simulink model "full_maneuver_single_veh"  (R2020a)
settings: Solver=VariableStepAuto  StartTime=0.0  StopTime=90  FixedStep=0.1  MaxStep=5e-2  RelTol=1e-3
InitFcn:
  | totalVehicles = 5;
  | if exist('vehStatesBus', 'var')==0
  | load vehBuses
  | end
  | if exist('vehErrorsBus', 'var')==0
  | load vehBuses
  | end
libraries: simulink x69, powerlib_meascontrol x6, autolibshared x6, dspsigops x3, eeGeneralControl x2
(part 1 of 6)
settings Model: Creator=fvall  LastModifiedBy=fvall
settings SFSimCC: CustomCodeUndefinedFunction=UseInterfaceOnly

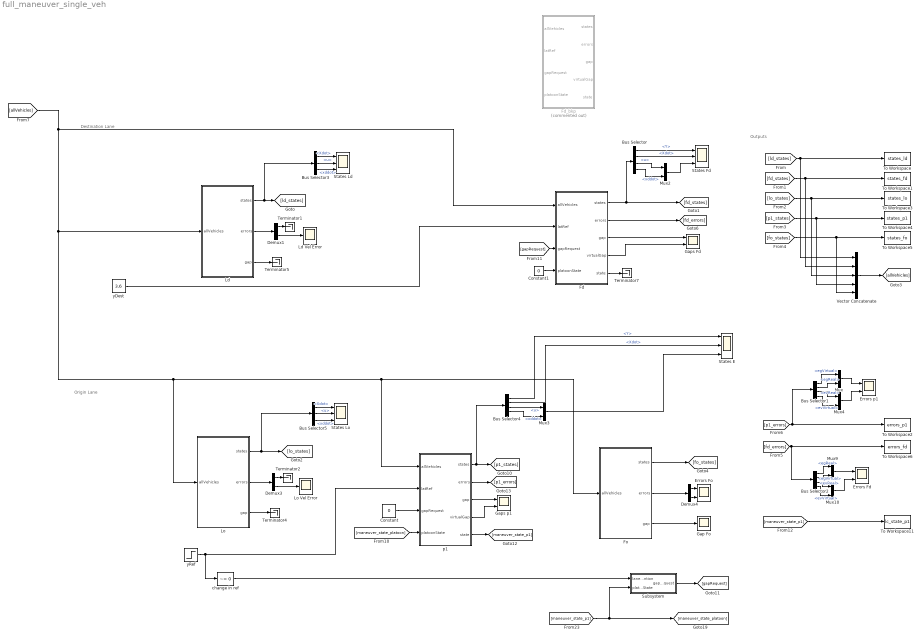
== system full_maneuver_single_veh ==
  note: Destination Lane
  note: Outputs
  note: Origin Lane
  Bus Selector : BusSelector  OutputSignals=Y,Xdot,u,xddot
  Bus Selector1 : BusSelector  OutputSignals=egVirtual,egReal,evReal,evVirtual
  Bus Selector2 : BusSelector  OutputSignals=egReal,egVirtual,evReal,evVirtual
  Bus Selector3 : BusSelector  OutputSignals=Xdot,u,xddot
  Bus Selector4 : BusSelector  OutputSignals=Y,Xdot,u,xddot
  Bus Selector5 : BusSelector  OutputSignals=Xdot,u,xddot
  Constant : Constant  Value=0
  Constant1 : Constant  Value=0
  Demux1 : Demux  Outputs=2
  Demux3 : Demux  Outputs=2
  Demux4 : Demux  Outputs=2
  Errors Fd : Scope  NumInputPorts=2
  Errors Fo : Scope  NumInputPorts=2
  Errors p1 : Scope  NumInputPorts=2
  Fd : Subsystem  mask{m=2000, lf=2.5, lr=2.5, maxAcceleration=3, minAcceleration=-8, maxJerk=50, minJerk=-50, maxDelta=0.43633, maxDeltaDot=0.16406, freeFlowVel=30, posInPlatoon=1, tau=0.5, A=[0 1 15 0;0 -3.06666666666667 0 -16.8666666666667;0 0 0 1;0 -0.933333333333333 0 -10.1333333333333], B=[0;24;0;36], C=[1 0 0 0;0 1 0 0;0 0 1 0;0 0 0 1], x0=24.5938, vx0=15, y0=3.6, h=0.56375, d0=0.5, minGapError=-100, maxGapError=Inf, velFilterGain=10, Kd=1.7738, Kp=0.17738, Ki=0, Ka=0.97561, Kdd=0.097561, velKi=0.0047047, velKp=0.093693, velKd=-0.53954, hFilterGain=1, hFilterSaturation=0.5, vMin=9.75, maxComfAccel=0.6, minComfAccel=-0.4, maxComfJerk=10, minComfJerk=-10, strategy=1, hLC=1.3256, d0LC=0.5, Klat=[0.0363636363636363 -0.0124557881655676 0.972727272727275 0.00274830322149061], L=[3 1 15 0;0 2.93333333333333 0 -16.8666666666667;0 0 12 1;0 -0.933333333333333 0 7.86666666666667]}
      mask prompts: m "autoblks_shared:autoblkVehBody3DofLat:blkPrm_m"; lf "autoblks_shared:autoblkVehBody3DofLat:blkPrm_a"; lr "autoblks_shared:autoblkVehBody3DofLat:blkPrm_b"; maxAcceleration "Max Acceleration"; minAcceleration "Min Acceleration"; maxJerk "Max Jerk"; minJerk "Min Jerk"; maxDelta "Max Delta"; maxDeltaDot "Max Delta Dot"; freeFlowVel "Free Flow Velocity"; posInPlatoon "Position in Platoon"; tau "Actuator Lag"; x0 "autoblks_shared:autoblkVehBody3DofLat:blkPrm_X_o"; vx0 "autoblks_shared:autoblkVehBody3DofLat:blkPrm_xdot_o"; y0 "autoblks_shared:autoblkVehBody3DofLat:blkPrm_Y_o"; h "Time Headway"; d0 "Standstill Gap"; minGapError "Min Gap Error"; maxGapError "Max Gap Error"; velFilterGain "Velocity Filter Gain"; hFilterGain "Headway Filter Gain"; hFilterSaturation "Headway Filter Saturation"; vMin "Min Velocity"; maxComfAccel "Max Comf Accel"; minComfAccel "Min Comf Accel"; maxComfJerk "Max Comf Jerk"; minComfJerk "Min Comf Jerk"; strategy "LC strategy"; hLC "Time Headway LC"; d0LC "Standstill Gap LC"; Klat "Lat Controller Gain"; L "Observer Gain"
      mask TypeOptions m: Vehicle Body 3DOF Single Track/m
      mask TypeOptions lf: Vehicle Body 3DOF Single Track/a
      mask TypeOptions lr: Vehicle Body 3DOF Single Track/b
      mask TypeOptions maxDelta: Lateral Control/Saturation/UpperLimit
      mask TypeOptions maxDeltaDot: Lateral Control/Rate Limiter/RisingSlewLimit
      mask TypeOptions posInPlatoon: posInPlatoon/Value
      mask TypeOptions A:
      | Lateral Control/Full State
      | Observer/Gain3/Gain
      mask TypeOptions B:
      | Lateral Control/Full State
      | Observer/Gain/Gain
      mask TypeOptions C:
      | Lateral Control/Full State
      | Observer/Gain1/Gain
      mask TypeOptions x0: Vehicle Body 3DOF Single Track/X_o
      mask TypeOptions vx0: Vehicle Body 3DOF Single Track/xdot_o
      mask TypeOptions y0: Vehicle Body 3DOF Single Track/Y_o
      mask TypeOptions strategy: strategy/Value
      mask TypeOptions Klat: Lateral Control/Gain1/Gain
      mask TypeOptions L:
      | Lateral Control/Full State
      | Observer/Gain2/Gain
      mask DialogControl DescGroupVar Prompt: 3DOF Vehicle with ACC
      mask DialogControl DescTextVar Prompt: Vehicle with ACC. The vehicle model is Simulink's 3DOF single track vehicle body. The controller is a PID with constant headway including headway error saturation and filtered leader velocity.
      mask DialogControl VehParams Prompt: Vehicle Parameters
      mask DialogControl m Prompt: Vehicle mass, m [kg]:
      mask DialogControl lf Prompt: Longitudinal distance from center of mass to front axle, a [m]:
      mask DialogControl lr Prompt: Longitudinal distance from center of mass to rear axle, b [m]:
      mask DialogControl latLinearModel Prompt: Lat Linear Model
      mask DialogControl InitStates Prompt: Initial State
      mask DialogControl x0 Prompt: Initial inertial frame longitudinal position, X_o [m]:
      mask DialogControl vx0 Prompt: Initial longitudinal velocity, xdot_o [m/s]:
      mask DialogControl y0 Prompt: Initial inertial frame lateral displacement, Y_o [m]:
      mask DialogControl Container3 Prompt: Veh Following Parameters
      mask DialogControl ComfortConstraints Prompt: Comfort Constraints
      mask DialogControl LCParams Prompt: Lane Change Params
  Fd_bkp : Subsystem  Commented=on  mask{m=2000, lf=2.5, lr=2.5, maxAcceleration=3, minAcceleration=-8, maxJerk=50, minJerk=-50, maxDelta=0.43633, maxDeltaDot=0.16406, freeFlowVel=30, posInPlatoon=1, tau=0.5, A=[0 1 20 0;0 -2.3 0 -21.4;0 0 0 1;0 -0.7 0 -7.6], B=[0;24;0;36], C=[1 0 0 0;0 1 0 0;0 0 1 0;0 0 0 1], x0=-6.2192, vx0=25, y0=3.6, h=0.56375, d0=0.32452, minHeadwayError=-100, maxHeadwayError=Inf, velFilterGain=10, Kd=1.7738, Kp=0.17738, Ki=0, Ka=0.97561, Kdd=0.097561, velKi=0.0019848, velKp=0.052702, velKd=-0.65465, hFilterGain=1, hFilterSaturation=0.5, vMin=16.25, maxComfAccel=0.6, minComfAccel=-0.4, maxComfJerk=10, minComfJerk=-10, strategy=1, hLC=1.9506, d0LC=0.32452, Klat=[0.0363636363636331 0.000980533179898461 1.32121212121203 0.0854574223245029], L=[3 1 20 0;0 3.7 0 -21.4;0 0 12 1;0 -0.7 0 10.4]}
      mask prompts: m "autoblks_shared:autoblkVehBody3DofLat:blkPrm_m"; lf "autoblks_shared:autoblkVehBody3DofLat:blkPrm_a"; lr "autoblks_shared:autoblkVehBody3DofLat:blkPrm_b"; maxAcceleration "Max Acceleration"; minAcceleration "Min Acceleration"; maxJerk "Max Jerk"; minJerk "Min Jerk"; maxDelta "Max Delta"; maxDeltaDot "Max Delta Dot"; freeFlowVel "Free Flow Velocity"; posInPlatoon "Position in Platoon"; tau "Actuator Lag"; x0 "autoblks_shared:autoblkVehBody3DofLat:blkPrm_X_o"; vx0 "autoblks_shared:autoblkVehBody3DofLat:blkPrm_xdot_o"; y0 "autoblks_shared:autoblkVehBody3DofLat:blkPrm_Y_o"; h "Time Headway"; d0 "Standstill Gap"; minHeadwayError "Min Headway Error"; maxHeadwayError "Max Headway Error"; velFilterGain "Velocity Filter Gain"; hFilterGain "Headway Filter Gain"; hFilterSaturation "Headway Filter Saturation"; vMin "Min Velocity"; maxComfAccel "Max Comf Accel"; minComfAccel "Min Comf Accel"; maxComfJerk "Max Comf Jerk"; minComfJerk "Min Comf Jerk"; strategy "LC strategy"; hLC "Time Headway LC"; d0LC "Standstill Gap LC"; Klat "Lat Controller Gain"; L "Observer Gain"
      mask TypeOptions m: Vehicle Body 3DOF Single Track/m
      mask TypeOptions lf: Vehicle Body 3DOF Single Track/a
      mask TypeOptions lr: Vehicle Body 3DOF Single Track/b
      mask TypeOptions maxDelta: Lateral Control/Saturation/UpperLimit
      mask TypeOptions maxDeltaDot: Lateral Control/Rate Limiter/RisingSlewLimit
      mask TypeOptions posInPlatoon: posInPlatoon/Value
      mask TypeOptions A:
      | Lateral Control/Full State
      | Observer/Gain3/Gain
      mask TypeOptions B:
      | Lateral Control/Full State
      | Observer/Gain/Gain
      mask TypeOptions C:
      | Lateral Control/Full State
      | Observer/Gain1/Gain
      mask TypeOptions x0: Vehicle Body 3DOF Single Track/X_o
      mask TypeOptions vx0: Vehicle Body 3DOF Single Track/xdot_o
      mask TypeOptions y0: Vehicle Body 3DOF Single Track/Y_o
      mask TypeOptions strategy: strategy/Value
      mask TypeOptions Klat: Lateral Control/Gain1/Gain
      mask TypeOptions L:
      | Lateral Control/Full State
      | Observer/Gain2/Gain
      mask DialogControl DescGroupVar Prompt: 3DOF Vehicle with ACC
      mask DialogControl DescTextVar Prompt: Vehicle with ACC. The vehicle model is Simulink's 3DOF single track vehicle body. The controller is a PID with constant headway including headway error saturation and filtered leader velocity.
      mask DialogControl VehParams Prompt: Vehicle Parameters
      mask DialogControl m Prompt: Vehicle mass, m [kg]:
      mask DialogControl lf Prompt: Longitudinal distance from center of mass to front axle, a [m]:
      mask DialogControl lr Prompt: Longitudinal distance from center of mass to rear axle, b [m]:
      mask DialogControl latLinearModel Prompt: Lat Linear Model
      mask DialogControl InitStates Prompt: Initial State
      mask DialogControl x0 Prompt: Initial inertial frame longitudinal position, X_o [m]:
      mask DialogControl vx0 Prompt: Initial longitudinal velocity, xdot_o [m/s]:
      mask DialogControl y0 Prompt: Initial inertial frame lateral displacement, Y_o [m]:
      mask DialogControl Container3 Prompt: Veh Following Parameters
      mask DialogControl ComfortConstraints Prompt: Comfort Constraints
      mask DialogControl LCParams Prompt: Lane Change Params
  Fo : Subsystem  mask{m=2000, lf=2.5, lr=2.5, maxAcceleration=3, minAcceleration=-8, maxJerk=50, minJerk=-50, freeFlowVel=30, tau=0.5, x0=0, vx0=20, y0=0, h=0.56375, d0=0.5, minGapError=-100, maxGapError=Inf, velFilterGain=10, Kd=1.7738, Kp=0.17738, Ki=0, Ka=0.97561, Kdd=0.097561, velKi=0.0047047, velKp=0.093693, velKd=-0.53954, hFilterGain=1, hFilterSaturation=0.5, vMin=13, maxComfAccel=0.6, minComfAccel=-0.4, maxComfJerk=10, minComfJerk=-10, hLC=1.6381, d0LC=0.5}
      mask prompts: m "autoblks_shared:autoblkVehBody3DofLat:blkPrm_m"; lf "autoblks_shared:autoblkVehBody3DofLat:blkPrm_a"; lr "autoblks_shared:autoblkVehBody3DofLat:blkPrm_b"; maxAcceleration "Max Acceleration"; minAcceleration "Min Acceleration"; maxJerk "Max Jerk"; minJerk "Min Jerk"; freeFlowVel "Free Flow Velocity"; tau "Actuator Lag"; x0 "autoblks_shared:autoblkVehBody3DofLat:blkPrm_X_o"; vx0 "autoblks_shared:autoblkVehBody3DofLat:blkPrm_xdot_o"; y0 "autoblks_shared:autoblkVehBody3DofLat:blkPrm_Y_o"; h "Time Headway"; d0 "Standstill Gap"; minGapError "Min Gap Error"; maxGapError "Max Gap Error"; velFilterGain "Velocity Filter Gain"; hFilterGain "Headway Filter Gain"; hFilterSaturation "Headway Filter Saturation"; vMin "Min Velocity"; maxComfAccel "Max Comf Accel"; minComfAccel "Min Comf Accel"; maxComfJerk "Max Comf Jerk"; minComfJerk "Min Comf Jerk"; hLC "Time Headway LC"; d0LC "Standstill Gap LC"
      mask TypeOptions m: Vehicle Body 3DOF Single Track/m
      mask TypeOptions lf: Vehicle Body 3DOF Single Track/a
      mask TypeOptions lr: Vehicle Body 3DOF Single Track/b
      mask TypeOptions x0: Vehicle Body 3DOF Single Track/X_o
      mask TypeOptions vx0: Vehicle Body 3DOF Single Track/xdot_o
      mask TypeOptions y0: Vehicle Body 3DOF Single Track/Y_o
      mask DialogControl DescGroupVar Prompt: 3DOF Vehicle with ACC
      mask DialogControl DescTextVar Prompt: Vehicle with ACC. The vehicle model is Simulink's 3DOF single track vehicle body. The controller is a PID with constant headway including headway error saturation and filtered leader velocity.
      mask DialogControl VehParams Prompt: Vehicle Parameters
      mask DialogControl m Prompt: Vehicle mass, m [kg]:
      mask DialogControl lf Prompt: Longitudinal distance from center of mass to front axle, a [m]:
      mask DialogControl lr Prompt: Longitudinal distance from center of mass to rear axle, b [m]:
      mask DialogControl InitStates Prompt: Initial State
      mask DialogControl x0 Prompt: Initial inertial frame longitudinal position, X_o [m]:
      mask DialogControl vx0 Prompt: Initial longitudinal velocity, xdot_o [m/s]:
      mask DialogControl y0 Prompt: Initial inertial frame lateral displacement, Y_o [m]:
      mask DialogControl Container3 Prompt: Veh Following Parameters
      mask DialogControl ComfortConstraints Prompt: Comfort Constraints
      mask DialogControl LaneChangeParams Prompt: Lane Change Params
  Gap Fo : Scope
  Gaps Fd : Scope  NumInputPorts=2
  Gaps p1 : Scope  NumInputPorts=2
  Ld : Subsystem  mask{m=2000, lf=2.5, lr=2.5, maxAcceleration=3, minAcceleration=-8, maxJerk=50, minJerk=-50, freeFlowVel=15, tau=0.5, x0=38.55, vx0=15, y0=3.6, h=0.56375, d0=0.5, minGapError=-100, maxGapError=Inf, velFilterGain=10, Kd=1.7738, Kp=0.17738, Ki=0, Ka=0.97561, Kdd=0.097561, velKi=0.0047047, velKp=0.093693, velKd=-0.53954, hFilterGain=1, hFilterSaturation=0.5, vMin=9.75, maxComfAccel=0.6, minComfAccel=-0.4, maxComfJerk=10, minComfJerk=-10, hLC=1.3256, d0LC=0.5}
      mask prompts: m "autoblks_shared:autoblkVehBody3DofLat:blkPrm_m"; lf "autoblks_shared:autoblkVehBody3DofLat:blkPrm_a"; lr "autoblks_shared:autoblkVehBody3DofLat:blkPrm_b"; maxAcceleration "Max Acceleration"; minAcceleration "Min Acceleration"; maxJerk "Max Jerk"; minJerk "Min Jerk"; freeFlowVel "Free Flow Velocity"; tau "Actuator Lag"; x0 "autoblks_shared:autoblkVehBody3DofLat:blkPrm_X_o"; vx0 "autoblks_shared:autoblkVehBody3DofLat:blkPrm_xdot_o"; y0 "autoblks_shared:autoblkVehBody3DofLat:blkPrm_Y_o"; h "Time Headway"; d0 "Standstill Gap"; minGapError "Min Gap Error"; maxGapError "Max Gap Error"; velFilterGain "Velocity Filter Gain"; hFilterGain "Headway Filter Gain"; hFilterSaturation "Headway Filter Saturation"; vMin "Min Velocity"; maxComfAccel "Max Comf Accel"; minComfAccel "Min Comf Accel"; maxComfJerk "Max Comf Jerk"; minComfJerk "Min Comf Jerk"; hLC "Time Headway LC"; d0LC "Standstill Gap LC"
      mask TypeOptions m: Vehicle Body 3DOF Single Track/m
      mask TypeOptions lf: Vehicle Body 3DOF Single Track/a
      mask TypeOptions lr: Vehicle Body 3DOF Single Track/b
      mask TypeOptions x0: Vehicle Body 3DOF Single Track/X_o
      mask TypeOptions vx0: Vehicle Body 3DOF Single Track/xdot_o
      mask TypeOptions y0: Vehicle Body 3DOF Single Track/Y_o
      mask DialogControl DescGroupVar Prompt: 3DOF Vehicle with ACC
      mask DialogControl DescTextVar Prompt: Vehicle with ACC. The vehicle model is Simulink's 3DOF single track vehicle body. The controller is a PID with constant headway including headway error saturation and filtered leader velocity.
      mask DialogControl VehParams Prompt: Vehicle Parameters
      mask DialogControl m Prompt: Vehicle mass, m [kg]:
      mask DialogControl lf Prompt: Longitudinal distance from center of mass to front axle, a [m]:
      mask DialogControl lr Prompt: Longitudinal distance from center of mass to rear axle, b [m]:
      mask DialogControl InitStates Prompt: Initial State
      mask DialogControl x0 Prompt: Initial inertial frame longitudinal position, X_o [m]:
      mask DialogControl vx0 Prompt: Initial longitudinal velocity, xdot_o [m/s]:
      mask DialogControl y0 Prompt: Initial inertial frame lateral displacement, Y_o [m]:
      mask DialogControl Container3 Prompt: Veh Following Parameters
      mask DialogControl ComfortConstraints Prompt: Comfort Constraints
      mask DialogControl LaneChangeParams Prompt: Lane Change Params
  Ld Vel Error : Scope
  Lo : Subsystem  mask{m=2000, lf=2.5, lr=2.5, maxAcceleration=3, minAcceleration=-8, maxJerk=50, minJerk=-50, freeFlowVel=20, tau=0.5, x0=33.55, vx0=20, y0=0, h=0.56375, d0=0.5, minGapError=-100, maxGapError=Inf, velFilterGain=10, Kd=1.7738, Kp=0.17738, Ki=0, Ka=0.97561, Kdd=0.097561, velKi=0.0047047, velKp=0.093693, velKd=-0.53954, hFilterGain=1, hFilterSaturation=0.5, vMin=13, maxComfAccel=0.6, minComfAccel=-0.4, maxComfJerk=10, minComfJerk=-10, hLC=1.6381, d0LC=0.5}
      mask prompts: m "autoblks_shared:autoblkVehBody3DofLat:blkPrm_m"; lf "autoblks_shared:autoblkVehBody3DofLat:blkPrm_a"; lr "autoblks_shared:autoblkVehBody3DofLat:blkPrm_b"; maxAcceleration "Max Acceleration"; minAcceleration "Min Acceleration"; maxJerk "Max Jerk"; minJerk "Min Jerk"; freeFlowVel "Free Flow Velocity"; tau "Actuator Lag"; x0 "autoblks_shared:autoblkVehBody3DofLat:blkPrm_X_o"; vx0 "autoblks_shared:autoblkVehBody3DofLat:blkPrm_xdot_o"; y0 "autoblks_shared:autoblkVehBody3DofLat:blkPrm_Y_o"; h "Time Headway"; d0 "Standstill Gap"; minGapError "Min Gap Error"; maxGapError "Max Gap Error"; velFilterGain "Velocity Filter Gain"; hFilterGain "Headway Filter Gain"; hFilterSaturation "Headway Filter Saturation"; vMin "Min Velocity"; maxComfAccel "Max Comf Accel"; minComfAccel "Min Comf Accel"; maxComfJerk "Max Comf Jerk"; minComfJerk "Min Comf Jerk"; hLC "Time Headway LC"; d0LC "Standstill Gap LC"
      mask TypeOptions m: Vehicle Body 3DOF Single Track/m
      mask TypeOptions lf: Vehicle Body 3DOF Single Track/a
      mask TypeOptions lr: Vehicle Body 3DOF Single Track/b
      mask TypeOptions x0: Vehicle Body 3DOF Single Track/X_o
      mask TypeOptions vx0: Vehicle Body 3DOF Single Track/xdot_o
      mask TypeOptions y0: Vehicle Body 3DOF Single Track/Y_o
      mask DialogControl DescGroupVar Prompt: 3DOF Vehicle with ACC
      mask DialogControl DescTextVar Prompt: Vehicle with ACC. The vehicle model is Simulink's 3DOF single track vehicle body. The controller is a PID with constant headway including headway error saturation and filtered leader velocity.
      mask DialogControl VehParams Prompt: Vehicle Parameters
      mask DialogControl m Prompt: Vehicle mass, m [kg]:
      mask DialogControl lf Prompt: Longitudinal distance from center of mass to front axle, a [m]:
      mask DialogControl lr Prompt: Longitudinal distance from center of mass to rear axle, b [m]:
      mask DialogControl InitStates Prompt: Initial State
      mask DialogControl x0 Prompt: Initial inertial frame longitudinal position, X_o [m]:
      mask DialogControl vx0 Prompt: Initial longitudinal velocity, xdot_o [m/s]:
      mask DialogControl y0 Prompt: Initial inertial frame lateral displacement, Y_o [m]:
      mask DialogControl Container3 Prompt: Veh Following Parameters
      mask DialogControl ComfortConstraints Prompt: Comfort Constraints
      mask DialogControl LaneChangeParams Prompt: Lane Change Params
  Lo Vel Error : Scope
  Mux{,2..4,9..10} (6 alike) : Mux  Inputs=2
  States E : Scope  NumInputPorts=3
  States Fd : Scope  NumInputPorts=3
  States Ld : Scope  NumInputPorts=3
  States Lo : Scope  NumInputPorts=3
  Subsystem : Subsystem
  Terminator{1..2,4..5,7} (5 alike) : Terminator
  To Workspace : ToWorkspace  VariableName=states_ld  SaveFormat=Timeseries  SampleTime=-1
  To Workspace1 : ToWorkspace  VariableName=states_fd  SaveFormat=Timeseries  SampleTime=-1
  To Workspace11 : ToWorkspace  VariableName=lc_state_p1  SaveFormat=Timeseries  SampleTime=-1
  To Workspace2 : ToWorkspace  VariableName=errors_p1  SaveFormat=Timeseries  SampleTime=-1
  To Workspace3 : ToWorkspace  VariableName=states_lo  SaveFormat=Timeseries  SampleTime=-1
  To Workspace4 : ToWorkspace  VariableName=states_p1  SaveFormat=Timeseries  SampleTime=-1
  To Workspace5 : ToWorkspace  VariableName=states_fo  SaveFormat=Timeseries  SampleTime=-1
  To Workspace6 : ToWorkspace  VariableName=errors_fd  SaveFormat=Timeseries  SampleTime=-1
  Vector Concatenate : Concatenate  NumInputs=5
  change in ref : simulink/Logic and Bit Operations/Compare To Constant  relop=~=  const=0  OutDataTypeStr=boolean
  p1 : Subsystem  mask{m=2000, lf=2.5, lr=2.5, maxAcceleration=3, minAcceleration=-8, maxJerk=50, minJerk=-50, maxDelta=0.43633, maxDeltaDot=0.16406, freeFlowVel=30, posInPlatoon=1, tau=0.5, A=[0 1 15 0;0 -3.06666666666667 0 -16.8666666666667;0 0 0 1;0 -0.933333333333333 0 -10.1333333333333], B=[0;24;0;36], C=[1 0 0 0;0 1 0 0;0 0 1 0;0 0 0 1], x0=16.775, vx0=20, y0=0, h=0.56375, d0=0.5, minGapError=-100, maxGapError=Inf, velFilterGain=10, Kd=1.7738, Kp=0.17738, Ki=0, Ka=0.97561, Kdd=0.097561, velKi=0.0047047, velKp=0.093693, velKd=-0.53954, hFilterGain=1, hFilterSaturation=0.5, vMin=13, maxComfAccel=0.6, minComfAccel=-0.4, maxComfJerk=10, minComfJerk=-10, strategy=1, hLC=1.6381, d0LC=0.5, Klat=[0.0363636363636363 -0.0124557881655676 0.972727272727275 0.00274830322149061], L=[3 1 15 0;0 2.93333333333333 0 -16.8666666666667;0 0 12 1;0 -0.933333333333333 0 7.86666666666667]}
      mask prompts: m "autoblks_shared:autoblkVehBody3DofLat:blkPrm_m"; lf "autoblks_shared:autoblkVehBody3DofLat:blkPrm_a"; lr "autoblks_shared:autoblkVehBody3DofLat:blkPrm_b"; maxAcceleration "Max Acceleration"; minAcceleration "Min Acceleration"; maxJerk "Max Jerk"; minJerk "Min Jerk"; maxDelta "Max Delta"; maxDeltaDot "Max Delta Dot"; freeFlowVel "Free Flow Velocity"; posInPlatoon "Position in Platoon"; tau "Actuator Lag"; x0 "autoblks_shared:autoblkVehBody3DofLat:blkPrm_X_o"; vx0 "autoblks_shared:autoblkVehBody3DofLat:blkPrm_xdot_o"; y0 "autoblks_shared:autoblkVehBody3DofLat:blkPrm_Y_o"; h "Time Headway"; d0 "Standstill Gap"; minGapError "Min Gap Error"; maxGapError "Max Gap Error"; velFilterGain "Velocity Filter Gain"; hFilterGain "Headway Filter Gain"; hFilterSaturation "Headway Filter Saturation"; vMin "Min Velocity"; maxComfAccel "Max Comf Accel"; minComfAccel "Min Comf Accel"; maxComfJerk "Max Comf Jerk"; minComfJerk "Min Comf Jerk"; strategy "LC strategy"; hLC "Time Headway LC"; d0LC "Standstill Gap LC"; Klat "Lat Controller Gain"; L "Observer Gain"
      mask TypeOptions m: Vehicle Body 3DOF Single Track/m
      mask TypeOptions lf: Vehicle Body 3DOF Single Track/a
      mask TypeOptions lr: Vehicle Body 3DOF Single Track/b
      mask TypeOptions maxDelta: Lateral Control/Saturation/UpperLimit
      mask TypeOptions maxDeltaDot: Lateral Control/Rate Limiter/RisingSlewLimit
      mask TypeOptions posInPlatoon: posInPlatoon/Value
      mask TypeOptions A:
      | Lateral Control/Full State
      | Observer/Gain3/Gain
      mask TypeOptions B:
      | Lateral Control/Full State
      | Observer/Gain/Gain
      mask TypeOptions C:
      | Lateral Control/Full State
      | Observer/Gain1/Gain
      mask TypeOptions x0: Vehicle Body 3DOF Single Track/X_o
      mask TypeOptions vx0: Vehicle Body 3DOF Single Track/xdot_o
      mask TypeOptions y0: Vehicle Body 3DOF Single Track/Y_o
      mask TypeOptions strategy: strategy/Value
      mask TypeOptions Klat: Lateral Control/Gain1/Gain
      mask TypeOptions L:
      | Lateral Control/Full State
      | Observer/Gain2/Gain
      mask DialogControl DescGroupVar Prompt: 3DOF Vehicle with ACC
      mask DialogControl DescTextVar Prompt: Vehicle with ACC. The vehicle model is Simulink's 3DOF single track vehicle body. The controller is a PID with constant headway including headway error saturation and filtered leader velocity.
      mask DialogControl VehParams Prompt: Vehicle Parameters
      mask DialogControl m Prompt: Vehicle mass, m [kg]:
      mask DialogControl lf Prompt: Longitudinal distance from center of mass to front axle, a [m]:
      mask DialogControl lr Prompt: Longitudinal distance from center of mass to rear axle, b [m]:
      mask DialogControl latLinearModel Prompt: Lat Linear Model
      mask DialogControl InitStates Prompt: Initial State
      mask DialogControl x0 Prompt: Initial inertial frame longitudinal position, X_o [m]:
      mask DialogControl vx0 Prompt: Initial longitudinal velocity, xdot_o [m/s]:
      mask DialogControl y0 Prompt: Initial inertial frame lateral displacement, Y_o [m]:
      mask DialogControl Container3 Prompt: Veh Following Parameters
      mask DialogControl ComfortConstraints Prompt: Comfort Constraints
      mask DialogControl LCParams Prompt: Lane Change Params
  yDest : Constant  Value=3.6
  yRef : Step  Time=2  After=3.6  SampleTime=0
  wires:
  Fd/2(errors) -> [fd_errors]
  [gapRequest] -> Fd/3(gapRequest)
  Constant1/1 -> Fd/4(platoonState)
  Constant/1 -> p1/3(gapRequest)
  [maneuver_state_platoon] -> p1/4(platoonState)
  Bus Selector/3 -> Mux2/1  "<u>"
  Bus Selector/2 -> States Fd/2  "<Xdot>"
  Fd/5(state) -> Terminator7/1
  Fd/4(virtualGap) -> Gaps Fd/2
  Fd/3(gap) -> Gaps Fd/1
  Demux3/2 -> Lo Vel Error/1
  Lo/3(gap) -> Terminator4/1
  Demux3/1 -> Terminator2/1
  Lo/2(errors) -> Demux3/1
  Bus Selector1/3 -> Mux4/1  "<evReal>"
  Bus Selector2/4 -> Mux10/2  "<evVirtual>"
  Ld/3(gap) -> Terminator5/1
  Bus Selector1/4 -> Mux4/2  "<evVirtual>"
  Mux/1 -> Errors p1/1
  Bus Selector2/1 -> Mux9/1  "<egReal>"
  Bus Selector4/3 -> Mux3/1  "<u>"
  Mux4/1 -> Errors p1/2
  Demux1/2 -> Ld Vel Error/1
  Ld/2(errors) -> Demux1/1
  Demux4/1 -> Errors Fo/1
  Bus Selector1/1 -> Mux/1  "<egVirtual>"
  [maneuver_state_p1] -> To Workspace11/1
  Bus Selector2/2 -> Mux9/2  "<egVirtual>"
  Fo/1(states) -> [fo_states]
  Bus Selector/1 -> States Fd/1  "<Y>"
  [maneuver_state_p1] -> Subsystem/2(platoonState), [maneuver_state_platoon]
  Fd/1(states) -> Bus Selector/1, [fd_states]
  Bus Selector1/2 -> Mux/2  "<egReal>"
  [ld_states] -> Vector Concatenate/1, To Workspace/1
  Bus Selector4/1 -> States E/1  "<Y>"
  yRef/1 -> p1/2(latRef), change in ref/1
  Bus Selector4/2 -> States E/2  "<Xdot>"
  Demux1/1 -> Terminator1/1
  [p1_errors] -> Bus Selector1/1, To Workspace2/1
  [allVehicles] -> Fd/1(allVehicles), Ld/1(allVehicles), Lo/1(allVehicles), p1/1(allVehicles), Fo/1(allVehicles)
  [p1_states] -> Vector Concatenate/4, To Workspace4/1
  [fo_states] -> Vector Concatenate/5, To Workspace5/1
  Demux4/2 -> Errors Fo/2
  [fd_errors] -> Bus Selector2/1, To Workspace6/1
  Mux10/1 -> Errors Fd/2
  Mux9/1 -> Errors Fd/1
  [lo_states] -> Vector Concatenate/3, To Workspace3/1
  change in ref/1 -> Subsystem/1(laneChangeIntention)
  Fo/2(errors) -> Demux4/1
  yDest/1 -> Fd/2(latRef)
  Fo/3(gap) -> Gap Fo/1
  [fd_states] -> Vector Concatenate/2, To Workspace1/1
  p1/2(errors) -> [p1_errors]
  Ld/1(states) -> Bus Selector3/1, [ld_states]
  p1/1(states) -> Bus Selector4/1, [p1_states]
  p1/3(gap) -> Gaps p1/1
  p1/5(state) -> [maneuver_state_p1]
  Vector Concatenate/1 -> [allVehicles]
  p1/4(virtualGap) -> Gaps p1/2
  Bus Selector2/3 -> Mux10/1  "<evReal>"
  Mux2/1 -> States Fd/3
  Bus Selector/4 -> Mux2/2  "<xddot>"
  Bus Selector4/4 -> Mux3/2  "<xddot>"
  Mux3/1 -> States E/3
  Subsystem/1(gapRequest) -> [gapRequest]
  Bus Selector3/1 -> States Ld/1  "<Xdot>"
  Bus Selector3/2 -> States Ld/2  "<u>"
  Bus Selector3/3 -> States Ld/3  "<xddot>"
  Bus Selector5/3 -> States Lo/3  "<xddot>"
  Bus Selector5/2 -> States Lo/2  "<u>"
  Bus Selector5/1 -> States Lo/1  "<Xdot>"
  Lo/1(states) -> Bus Selector5/1, [lo_states]

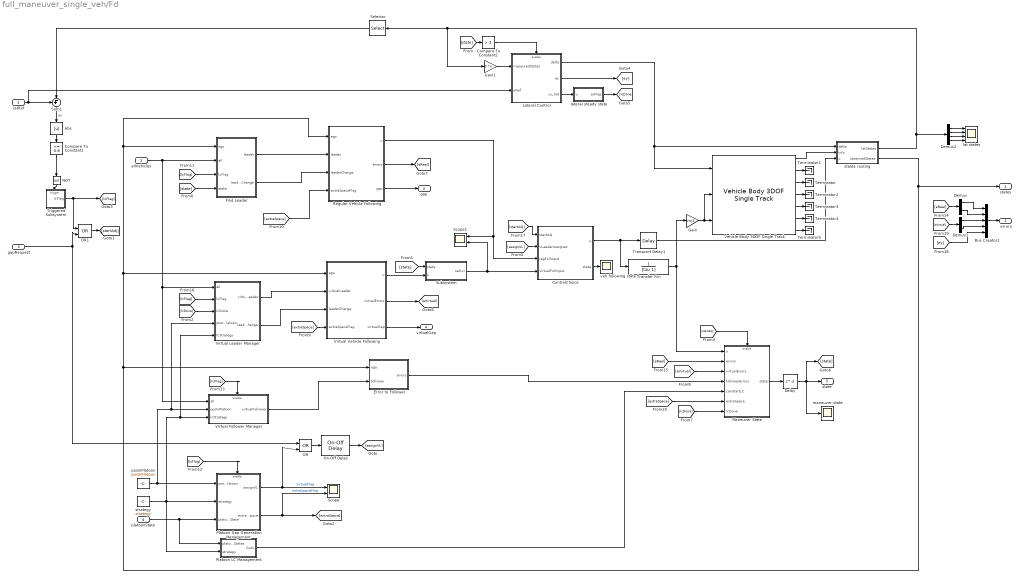
== system full_maneuver_single_veh/Fd ==
  allVehicles : Inport
  latRef : Inport  Port=2
  gapRequest : Inport  Port=3
  platoonState : Inport  Port=4
  Abs : Abs
  Bus Creator1 : BusCreator  Inputs=5  OutDataTypeStr=Bus: vehErrorsBus  NonVirtualBus=on
      settings: InheritFromInputs=off
  Compare To Constant1 : simulink/Logic and Bit Operations/Compare To Constant  relop=<=  const=0.8  OutDataTypeStr=boolean
  Compare To Constant2 : simulink/Logic and Bit Operations/Compare To Constant  relop=>  const=3  OutDataTypeStr=boolean
  ControlChoice : Stateflow chart  TreatAsAtomicUnit=on
  Delay : Delay
  Demux : Demux  Outputs=2
  Demux1 : Demux  Outputs=2
  Demux2 : Demux
  Error to Follower : Subsystem
  Find Leader : Subsystem
  Gain : Gain  Gain=m/2
  Gain1 : Gain  Gain=C  Multiplication=Matrix(K*u)
  Lateral Control : Subsystem
  Maneuver State : Subsystem
  NOT : Logic  Operator=NOT  IconShape=distinctive  AllPortsSameDT=off  OutDataTypeStr=boolean
  OR : Logic  Operator=OR  IconShape=distinctive  AllPortsSameDT=off  OutDataTypeStr=boolean
  OR1 : Logic  Operator=OR  IconShape=distinctive  AllPortsSameDT=off  OutDataTypeStr=boolean
  On-Off Delay : eeGeneralControl/On-Off Delay  LabelModeActiveChoice=Continuous  Td_on=0.1  Td_off=1  IC=0  Ts=0
      settings: SourceProductBaseCode=PS
  Platoon Gap Generation Management : Subsystem
  Platoon LC Management : Subsystem
  Regular Vehicle Following : Subsystem
  Scope : Scope  NumInputPorts=2
  Scope1 : Scope  NumInputPorts=2
  Selector : Selector  InputPortWidth=4  IndexOptions=Index vector (dialog)  Indices=1  OutputSizes=1
  Subsystem : Subsystem
  Sum1 : Sum  Inputs=+-|
  Terminator{,1..5} (6 alike) : Terminator
  Transfer Fcn : TransferFcn  Denominator=[tau 1]
  Transport Delay1 : TransportDelay  DelayTime=0.01
  Triggered Subsystem : Subsystem  TreatAsAtomicUnit=on
  Vehicle Body 3DOF Single Track : autolibshared/Vehicle Body 3DOF Single Track  trackMode=Single (bicycle)  inputMode=External longitudinal forces  frontSteerMode=on  rearSteerMode=off  windMode=off  muMode=off  extFMode=off  extMMode=off  extXo=off  extpsio=off  extxdoto=off  extro=off  extYo=off  extTamb=off  extydoto=off  aMode=2  NF=2  NR=2  m=m  a=lf  b=lr  h=0.35  X_o=x0  xdot_o=vx0  CalphaMode=off  sigmaMode=on  d=0  w=[1.4,1.4]  Cy_f=12e3  Cy_r=11e3  sigma_f=.1  sigma_r=.1  alpha_f_brk=[-.1 .1]  Cy_f_data=[-9e3 9e3]  alpha_r_brk=[-.1 .1]  Cy_r_data=[-9e3 9e3]  Y_o=y0  ydot_o=0  Izz=4000  psi_o=0  r_o=0  Af=2  Cd=.3  Cl=.1  Cpm=.1  beta_w=[0:0.01:0.3]  Cs=[0:0.03:0.9]  Cym=[0:0.01:0.3]  Pabs=101325  Tair=273  g=9.81  mu=1  xdot_tol=.01  Fznom=5000  Fxtire_sat=7e4  Fytire_sat=7e4  longOff=0  latOff=0  vertOff=0  wrapAng=off
      settings: SourceProductBaseCode=PW,MT,VE,VP
  Virtual Follower Manager : Subsystem  TreatAsAtomicUnit=on
  Virtual Leader Manager : Subsystem  TreatAsAtomicUnit=on
  Virtual Vehicle Following : Subsystem  TreatAsAtomicUnit=on
  lat states : Scope  NumInputPorts=4
  lateral steady state : Subsystem
  maneuver state : Scope
  posInPlatoon : Constant  Value=posInPlatoon
  states routing : Subsystem
  strategy : Constant  Value=strategy
  veh following state : Scope
  states : Outport  VectorParamsAs1DForOutWhenUnconnected=off
  errors : Outport  Port=2  VectorParamsAs1DForOutWhenUnconnected=off
  gap : Outport  Port=3  VectorParamsAs1DForOutWhenUnconnected=off
  virtualGap : Outport  Port=4  VectorParamsAs1DForOutWhenUnconnected=off
  state : Outport  Port=5  VectorParamsAs1DForOutWhenUnconnected=off
  wires:
  On-Off Delay/1 -> [assignVL]
  Transport Delay1/1 -> states routing/3(u)
  ControlChoice/2(state) -> veh following state/1
  Virtual Follower Manager/1(virtualFollower) -> Error to Follower/2(follower)
  ControlChoice/1(u) -> Transport Delay1/1, Transfer Fcn/1
  Vehicle Body 3DOF Single Track/7 -> Terminator5/1
  Vehicle Body 3DOF Single Track/6 -> Terminator4/1
  Vehicle Body 3DOF Single Track/5 -> Terminator3/1
  Vehicle Body 3DOF Single Track/4 -> Terminator2/1
  Vehicle Body 3DOF Single Track/2 -> Terminator1/1
  Selector/1 -> Sum1/2
  Demux2/4 -> lat states/4
  Demux2/3 -> lat states/3
  Demux2/2 -> lat states/2
  Demux2/1 -> lat states/1
  Lateral Control/1(delta) -> states routing/1(delta), Vehicle Body 3DOF Single Track/1
  OR/1 -> On-Off Delay/1
  Bus Creator1/1 -> errors/1
  [ey] -> Bus Creator1/5
  Demux1/2 -> Bus Creator1/4
  Demux1/1 -> Bus Creator1/3
  Demux/2 -> Bus Creator1/2
  Demux/1 -> Bus Creator1/1
  [eReal] -> Demux/1
  [eVirtual] -> Demux1/1
  Lateral Control/2(ey) -> [ey]
  lateral steady state/1(ssFlag) -> [lcDone]
  Lateral Control/3(vy_hat) -> lateral steady state/1(u)
  NOT/1 -> Triggered Subsystem/Trigger
  Gain1/1 -> Lateral Control/1(measuredStates)
  states routing/1(latStates) -> Gain1/1, Selector/1, Demux2/1
  OR1/1 -> [startAdj]
  [state] -> Find Leader/4(state)
  strategy/1 -> Platoon Gap Generation Management/2(strategy), Platoon LC Management/2(strategy), Virtual Follower Manager/3(lcStrategy), Virtual Leader Manager/5(lcStrategy)
  Delay/1 -> maneuver state/1, [state], state/1
  platoonState/1 -> Platoon LC Management/1(platoonStates), Platoon Gap Generation Management/3(platoonState)
  [state] -> Compare To Constant2/1
  Virtual Vehicle Following/3(virtualGap) -> virtualGap/1
  Compare To Constant2/1 -> Lateral Control/Enable
  Virtual Vehicle Following/1(u) -> Subsystem/2(u)
  Regular Vehicle Following/1(u) -> Scope1/1, ControlChoice/3(regFollInput)
  Regular Vehicle Following/3(gap) -> gap/1
  allVehicles/1 -> Virtual Follower Manager/1(all), Virtual Leader Manager/1(all), Find Leader/2(all)
  Abs/1 -> Compare To Constant1/1
  Platoon Gap Generation Management/2(extraSpace) -> [extraSpace], Scope/2  "extraSpaceFlag"
  Gain/1 -> Vehicle Body 3DOF Single Track/2, Vehicle Body 3DOF Single Track/3
  Vehicle Body 3DOF Single Track/1 -> states routing/2(Info)
  Vehicle Body 3DOF Single Track/3 -> Terminator/1
  latRef/1 -> Sum1/1, Lateral Control/2(yRef)
  states routing/2(observedStates) -> Error to Follower/1(ego), Find Leader/1(ego), Regular Vehicle Following/1(ego), Virtual Vehicle Following/1(ego), states/1
  Transfer Fcn/1 -> Maneuver State/1(u), Gain/1
  Sum1/1 -> Abs/1  "ey"
  Find Leader/2(leaderChange) -> Regular Vehicle Following/3(leaderChange)
  Subsystem/1(sat(u)) -> Scope1/2, ControlChoice/4(virtualFollInput)
  Find Leader/1(leader) -> Regular Vehicle Following/2(leader)
  [state] -> Subsystem/1(state)
  posInPlatoon/1 -> Platoon Gap Generation Management/1(posInPlatoon), Virtual Follower Manager/2(posInPlatoon), Virtual Leader Manager/4(posInPlatoon)
  Virtual Leader Manager/1(virtualLeader) -> Virtual Vehicle Following/2(virtualLeader)
  [startAdj] -> ControlChoice/1(startAdj)
  Compare To Constant1/1 -> NOT/1
  Virtual Leader Manager/2(leaderChange) -> Virtual Vehicle Following/3(leaderChange)
  Virtual Vehicle Following/2(virtualErrors) -> [eVirtual]
  Regular Vehicle Following/2(errors) -> [eReal]
  Triggered Subsystem/1(lcFlag) -> OR1/1, [lcFlag]
  gapRequest/1 -> OR1/2, OR/1
  [assignVL] -> ControlChoice/2(vLeaderAssigned)
  Platoon Gap Generation Management/1(assignVL) -> Scope/1, OR/2  "virtualFlag"
  [extraSpace] -> Virtual Vehicle Following/4(extraSpaceFlag)
  [extraSpace] -> Regular Vehicle Following/4(extraSpaceFlag)
  [lcFlag] -> Find Leader/3(lcFlag)
  [lcFlag] -> Platoon Gap Generation Management/Enable
  [lcFlag] -> Virtual Follower Manager/Enable
  [lcDone] -> Virtual Leader Manager/3(lcDone)
  [lcFlag] -> Virtual Leader Manager/2(lcFlag)
  Maneuver State/1(state) -> Delay/1
  Error to Follower/1(errors) -> Maneuver State/4(followerErrors)
  Platoon LC Management/1(Out1) -> Maneuver State/5(canStartLC)
  [startAdj] -> Maneuver State/Enable
  [lcDone] -> Maneuver State/7(lcDone)
  [eVirtual] -> Maneuver State/3(virtualErrors)
  [eReal] -> Maneuver State/2(errors)
  [extraSpace] -> Maneuver State/6(extraSpace)

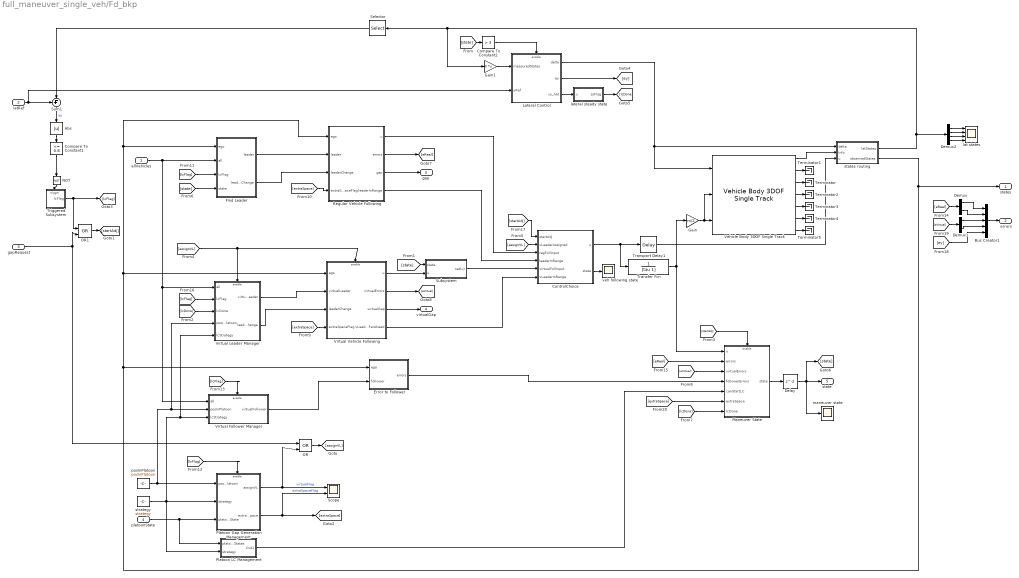
== system full_maneuver_single_veh/Fd_bkp ==
  allVehicles : Inport
  latRef : Inport  Port=2
  gapRequest : Inport  Port=3
  platoonState : Inport  Port=4
  Abs : Abs
  Bus Creator1 : BusCreator  Inputs=5  OutDataTypeStr=Bus: vehErrorsBus  NonVirtualBus=on
      settings: InheritFromInputs=off
  Compare To Constant1 : simulink/Logic and Bit Operations/Compare To Constant  relop=<=  const=0.8  OutDataTypeStr=boolean
  Compare To Constant2 : simulink/Logic and Bit Operations/Compare To Constant  relop=>  const=3  OutDataTypeStr=boolean
  ControlChoice : Stateflow chart  TreatAsAtomicUnit=on
  Delay : Delay
  Demux : Demux  Outputs=2
  Demux1 : Demux  Outputs=2
  Demux2 : Demux
  Error to Follower : Subsystem
  Find Leader : Subsystem
  Gain : Gain  Gain=m/2
  Gain1 : Gain  Gain=C  Multiplication=Matrix(K*u)
  Lateral Control : Subsystem
  Maneuver State : Subsystem
  NOT : Logic  Operator=NOT  IconShape=distinctive  AllPortsSameDT=off  OutDataTypeStr=boolean
  OR : Logic  Operator=OR  IconShape=distinctive  AllPortsSameDT=off  OutDataTypeStr=boolean
  OR1 : Logic  Operator=OR  IconShape=distinctive  AllPortsSameDT=off  OutDataTypeStr=boolean
  Platoon Gap Generation Management : Subsystem
  Platoon LC Management : Subsystem
  Regular Vehicle Following : Subsystem
  Scope : Scope  NumInputPorts=2
  Selector : Selector  InputPortWidth=4  IndexOptions=Index vector (dialog)  Indices=1  OutputSizes=1
  Subsystem : Subsystem
  Sum1 : Sum  Inputs=+-|
  Terminator{,1..5} (6 alike) : Terminator
  Transfer Fcn : TransferFcn  Denominator=[tau 1]
  Transport Delay1 : TransportDelay  DelayTime=0.01
  Triggered Subsystem : Subsystem  TreatAsAtomicUnit=on
  Vehicle Body 3DOF Single Track : autolibshared/Vehicle Body 3DOF Single Track  trackMode=Single (bicycle)  inputMode=External longitudinal forces  frontSteerMode=on  rearSteerMode=off  windMode=off  muMode=off  extFMode=off  extMMode=off  extXo=off  extpsio=off  extxdoto=off  extro=off  extYo=off  extTamb=off  extydoto=off  aMode=2  NF=2  NR=2  m=m  a=lf  b=lr  h=0.35  X_o=x0  xdot_o=vx0  CalphaMode=off  sigmaMode=on  d=0  w=[1.4,1.4]  Cy_f=12e3  Cy_r=11e3  sigma_f=.1  sigma_r=.1  alpha_f_brk=[-.1 .1]  Cy_f_data=[-9e3 9e3]  alpha_r_brk=[-.1 .1]  Cy_r_data=[-9e3 9e3]  Y_o=y0  ydot_o=0  Izz=4000  psi_o=0  r_o=0  Af=2  Cd=.3  Cl=.1  Cpm=.1  beta_w=[0:0.01:0.3]  Cs=[0:0.03:0.9]  Cym=[0:0.01:0.3]  Pabs=101325  Tair=273  g=9.81  mu=1  xdot_tol=.01  Fznom=5000  Fxtire_sat=7e4  Fytire_sat=7e4  longOff=0  latOff=0  vertOff=0  wrapAng=off
      settings: SourceProductBaseCode=PW,MT,VE,VP
  Virtual Follower Manager : Subsystem  TreatAsAtomicUnit=on
  Virtual Leader Manager : Subsystem  TreatAsAtomicUnit=on
  Virtual Vehicle Following : Subsystem  TreatAsAtomicUnit=on
  lat states : Scope  NumInputPorts=4
  lateral steady state : Subsystem
  maneuver state : Scope
  posInPlatoon : Constant  Value=posInPlatoon
  states routing : Subsystem
  strategy : Constant  Value=strategy
  veh following state : Scope
  states : Outport  VectorParamsAs1DForOutWhenUnconnected=off
  errors : Outport  Port=2  VectorParamsAs1DForOutWhenUnconnected=off
  gap : Outport  Port=3  VectorParamsAs1DForOutWhenUnconnected=off
  virtualGap : Outport  Port=4  VectorParamsAs1DForOutWhenUnconnected=off
  state : Outport  Port=5  VectorParamsAs1DForOutWhenUnconnected=off
  wires:
  Transport Delay1/1 -> states routing/3(u)
  ControlChoice/2(state) -> veh following state/1
  Virtual Follower Manager/1(virtualFollower) -> Error to Follower/2(follower)
  ControlChoice/1(u) -> Transport Delay1/1, Transfer Fcn/1
  Vehicle Body 3DOF Single Track/7 -> Terminator5/1
  Vehicle Body 3DOF Single Track/6 -> Terminator4/1
  Vehicle Body 3DOF Single Track/5 -> Terminator3/1
  Vehicle Body 3DOF Single Track/4 -> Terminator2/1
  Vehicle Body 3DOF Single Track/2 -> Terminator1/1
  Selector/1 -> Sum1/2
  Demux2/4 -> lat states/4
  Demux2/3 -> lat states/3
  Demux2/2 -> lat states/2
  Demux2/1 -> lat states/1
  Lateral Control/1(delta) -> states routing/1(delta), Vehicle Body 3DOF Single Track/1
  OR/1 -> [assignVL]
  Bus Creator1/1 -> errors/1
  [ey] -> Bus Creator1/5
  Demux1/2 -> Bus Creator1/4
  Demux1/1 -> Bus Creator1/3
  Demux/2 -> Bus Creator1/2
  Demux/1 -> Bus Creator1/1
  [eReal] -> Demux/1
  [eVirtual] -> Demux1/1
  Lateral Control/2(ey) -> [ey]
  lateral steady state/1(ssFlag) -> [lcDone]
  Lateral Control/3(vy_hat) -> lateral steady state/1(u)
  NOT/1 -> Triggered Subsystem/Trigger
  Gain1/1 -> Lateral Control/1(measuredStates)
  states routing/1(latStates) -> Gain1/1, Selector/1, Demux2/1
  OR1/1 -> [startAdj]
  Virtual Vehicle Following/4(vLeaderFarAhead) -> ControlChoice/6(vLeaderInRange)
  [state] -> Find Leader/4(state)
  strategy/1 -> Platoon Gap Generation Management/2(strategy), Platoon LC Management/2(strategy), Virtual Follower Manager/3(lcStrategy), Virtual Leader Manager/5(lcStrategy)
  Delay/1 -> maneuver state/1, [state], state/1
  platoonState/1 -> Platoon LC Management/1(platoonStates), Platoon Gap Generation Management/3(platoonState)
  [state] -> Compare To Constant2/1
  Virtual Vehicle Following/3(virtualGap) -> virtualGap/1
  Compare To Constant2/1 -> Lateral Control/Enable
  Virtual Vehicle Following/1(u) -> Subsystem/2(u)
  Regular Vehicle Following/1(u) -> ControlChoice/3(regFollInput)
  Regular Vehicle Following/3(gap) -> gap/1
  allVehicles/1 -> Virtual Follower Manager/1(all), Virtual Leader Manager/1(all), Find Leader/2(all)
  Abs/1 -> Compare To Constant1/1
  Platoon Gap Generation Management/2(extraSpace) -> [extraSpace], Scope/2  "extraSpaceFlag"
  Gain/1 -> Vehicle Body 3DOF Single Track/2, Vehicle Body 3DOF Single Track/3
  Vehicle Body 3DOF Single Track/1 -> states routing/2(Info)
  Vehicle Body 3DOF Single Track/3 -> Terminator/1
  latRef/1 -> Sum1/1, Lateral Control/2(yRef)
  states routing/2(observedStates) -> Error to Follower/1(ego), Find Leader/1(ego), Regular Vehicle Following/1(ego), Virtual Vehicle Following/1(ego), states/1
  Transfer Fcn/1 -> Maneuver State/1(u), Gain/1
  Sum1/1 -> Abs/1  "ey"
  Find Leader/2(leaderChange) -> Regular Vehicle Following/3(leaderChange)
  Subsystem/1(sat(u)) -> ControlChoice/5(virtualFollInput)
  Regular Vehicle Following/4(leaderInRange) -> ControlChoice/4(leaderInRange)
  Find Leader/1(leader) -> Regular Vehicle Following/2(leader)
  [state] -> Subsystem/1(state)
  posInPlatoon/1 -> Platoon Gap Generation Management/1(posInPlatoon), Virtual Follower Manager/2(posInPlatoon), Virtual Leader Manager/4(posInPlatoon)
  Virtual Leader Manager/1(virtualLeader) -> Virtual Vehicle Following/2(virtualLeader)
  [startAdj] -> ControlChoice/1(startAdj)
  Compare To Constant1/1 -> NOT/1
  Virtual Leader Manager/2(leaderChange) -> Virtual Vehicle Following/3(leaderChange)
  Virtual Vehicle Following/2(virtualErrors) -> [eVirtual]
  Regular Vehicle Following/2(errors) -> [eReal]
  Triggered Subsystem/1(lcFlag) -> OR1/1, [lcFlag]
  gapRequest/1 -> OR1/2, OR/1
  [assignVL] -> Virtual Leader Manager/Enable, Virtual Vehicle Following/Enable
  [assignVL] -> ControlChoice/2(vLeaderAssigned)
  Platoon Gap Generation Management/1(assignVL) -> Scope/1, OR/2  "virtualFlag"
  [extraSpace] -> Virtual Vehicle Following/4(extraSpaceFlag)
  [extraSpace] -> Regular Vehicle Following/4(extraSpaceFlag)
  [lcFlag] -> Find Leader/3(lcFlag)
  [lcFlag] -> Platoon Gap Generation Management/Enable
  [lcFlag] -> Virtual Follower Manager/Enable
  [lcDone] -> Virtual Leader Manager/3(lcDone)
  [lcFlag] -> Virtual Leader Manager/2(lcFlag)
  Maneuver State/1(state) -> Delay/1
  Error to Follower/1(errors) -> Maneuver State/4(followerErrors)
  Platoon LC Management/1(Out1) -> Maneuver State/5(canStartLC)
  [startAdj] -> Maneuver State/Enable
  [lcDone] -> Maneuver State/7(lcDone)
  [eVirtual] -> Maneuver State/3(virtualErrors)
  [eReal] -> Maneuver State/2(errors)
  [extraSpace] -> Maneuver State/6(extraSpace)

== system full_maneuver_single_veh/Fo ==
  allVehicles : Inport
  Constant{,1,3,6} (4 alike) : Constant  Value=0
  Gain : Gain  Gain=m/2
  Regular Vehicle Following : Subsystem
  Terminator{,1..3,9..12} (8 alike) : Terminator
  Transfer Fcn : TransferFcn  Denominator=[tau 1]
  Transport Delay1 : TransportDelay  DelayTime=0.01
  Vehicle Body 3DOF Single Track : autolibshared/Vehicle Body 3DOF Single Track  trackMode=Single (bicycle)  inputMode=External longitudinal forces  frontSteerMode=on  rearSteerMode=off  windMode=off  muMode=off  extFMode=off  extMMode=off  extXo=off  extpsio=off  extxdoto=off  extro=off  extYo=off  extTamb=off  extydoto=off  aMode=2  NF=2  NR=2  m=m  a=lf  b=lr  h=0.35  X_o=x0  xdot_o=vx0  CalphaMode=off  sigmaMode=on  d=0  w=[1.4,1.4]  Cy_f=12e3  Cy_r=11e3  sigma_f=.1  sigma_r=.1  alpha_f_brk=[-.1 .1]  Cy_f_data=[-9e3 9e3]  alpha_r_brk=[-.1 .1]  Cy_r_data=[-9e3 9e3]  Y_o=y0  ydot_o=0  Izz=4000  psi_o=0  r_o=0  Af=2  Cd=.3  Cl=.1  Cpm=.1  beta_w=[0:0.01:0.3]  Cs=[0:0.03:0.9]  Cym=[0:0.01:0.3]  Pabs=101325  Tair=273  g=9.81  mu=1  xdot_tol=.01  Fznom=5000  Fxtire_sat=7e4  Fytire_sat=7e4  longOff=0  latOff=0  vertOff=0  wrapAng=off
      settings: SourceProductBaseCode=PW,MT,VE,VP
  findLeader : Subsystem
  states routing : Subsystem
  states : Outport  VectorParamsAs1DForOutWhenUnconnected=off
  errors : Outport  Port=2  VectorParamsAs1DForOutWhenUnconnected=off
  gap : Outport  Port=3  VectorParamsAs1DForOutWhenUnconnected=off
  wires:
  Vehicle Body 3DOF Single Track/4 -> Terminator9/1
  Vehicle Body 3DOF Single Track/7 -> Terminator12/1
  Vehicle Body 3DOF Single Track/6 -> Terminator11/1
  Vehicle Body 3DOF Single Track/3 -> Terminator/1
  Vehicle Body 3DOF Single Track/5 -> Terminator10/1
  Vehicle Body 3DOF Single Track/2 -> Terminator2/1
  states routing/1(latStates) -> Terminator1/1
  Constant6/1 -> findLeader/3(lcFlag)
  Constant1/1 -> findLeader/4(state)
  Regular Vehicle Following/3(gap) -> gap/1
  allVehicles/1 -> findLeader/2(all)
  Gain/1 -> Vehicle Body 3DOF Single Track/2, Vehicle Body 3DOF Single Track/3
  Vehicle Body 3DOF Single Track/1 -> states routing/2(Info)
  states routing/2(observedStates) -> states/1, findLeader/1(ego), Regular Vehicle Following/1(ego)
  Transport Delay1/1 -> Transfer Fcn/1, states routing/3(u)
  findLeader/2(leaderChange) -> Regular Vehicle Following/3(leaderChange)
  Regular Vehicle Following/1(u) -> Transport Delay1/1  "u"
  Regular Vehicle Following/2(errors) -> errors/1
  Constant/1 -> Vehicle Body 3DOF Single Track/1, states routing/1(delta)  "delta"
  Constant3/1 -> Regular Vehicle Following/4(extraSpaceFlag)
  Regular Vehicle Following/4(leaderInRange) -> Terminator3/1
  findLeader/1(leader) -> Regular Vehicle Following/2(leader)
  Transfer Fcn/1 -> Gain/1

== system full_maneuver_single_veh/Ld ==
  allVehicles : Inport
  Constant{,1,3,6} (4 alike) : Constant  Value=0
  Gain : Gain  Gain=m/2
  Regular Vehicle Following : Subsystem
  Terminator{,1..3,9..12} (8 alike) : Terminator
  Transfer Fcn : TransferFcn  Denominator=[tau 1]
  Transport Delay1 : TransportDelay  DelayTime=0.01
  Vehicle Body 3DOF Single Track : autolibshared/Vehicle Body 3DOF Single Track  trackMode=Single (bicycle)  inputMode=External longitudinal forces  frontSteerMode=on  rearSteerMode=off  windMode=off  muMode=off  extFMode=off  extMMode=off  extXo=off  extpsio=off  extxdoto=off  extro=off  extYo=off  extTamb=off  extydoto=off  aMode=2  NF=2  NR=2  m=m  a=lf  b=lr  h=0.35  X_o=x0  xdot_o=vx0  CalphaMode=off  sigmaMode=on  d=0  w=[1.4,1.4]  Cy_f=12e3  Cy_r=11e3  sigma_f=.1  sigma_r=.1  alpha_f_brk=[-.1 .1]  Cy_f_data=[-9e3 9e3]  alpha_r_brk=[-.1 .1]  Cy_r_data=[-9e3 9e3]  Y_o=y0  ydot_o=0  Izz=4000  psi_o=0  r_o=0  Af=2  Cd=.3  Cl=.1  Cpm=.1  beta_w=[0:0.01:0.3]  Cs=[0:0.03:0.9]  Cym=[0:0.01:0.3]  Pabs=101325  Tair=273  g=9.81  mu=1  xdot_tol=.01  Fznom=5000  Fxtire_sat=7e4  Fytire_sat=7e4  longOff=0  latOff=0  vertOff=0  wrapAng=off
      settings: SourceProductBaseCode=PW,MT,VE,VP
  findLeader : Subsystem
  states routing : Subsystem
  states : Outport  VectorParamsAs1DForOutWhenUnconnected=off
  errors : Outport  Port=2  VectorParamsAs1DForOutWhenUnconnected=off
  gap : Outport  Port=3  VectorParamsAs1DForOutWhenUnconnected=off
  wires:
  Vehicle Body 3DOF Single Track/4 -> Terminator9/1
  Vehicle Body 3DOF Single Track/7 -> Terminator12/1
  Vehicle Body 3DOF Single Track/6 -> Terminator11/1
  Vehicle Body 3DOF Single Track/3 -> Terminator/1
  Vehicle Body 3DOF Single Track/5 -> Terminator10/1
  Vehicle Body 3DOF Single Track/2 -> Terminator2/1
  states routing/1(latStates) -> Terminator1/1
  Constant6/1 -> findLeader/3(lcFlag)
  Constant1/1 -> findLeader/4(state)
  Regular Vehicle Following/3(gap) -> gap/1
  allVehicles/1 -> findLeader/2(all)
  Gain/1 -> Vehicle Body 3DOF Single Track/2, Vehicle Body 3DOF Single Track/3
  Vehicle Body 3DOF Single Track/1 -> states routing/2(Info)
  states routing/2(observedStates) -> states/1, findLeader/1(ego), Regular Vehicle Following/1(ego)
  Transport Delay1/1 -> Transfer Fcn/1, states routing/3(u)
  findLeader/2(leaderChange) -> Regular Vehicle Following/3(leaderChange)
  Regular Vehicle Following/1(u) -> Transport Delay1/1  "u"
  Regular Vehicle Following/2(errors) -> errors/1
  Constant/1 -> Vehicle Body 3DOF Single Track/1, states routing/1(delta)  "delta"
  Constant3/1 -> Regular Vehicle Following/4(extraSpaceFlag)
  Regular Vehicle Following/4(leaderInRange) -> Terminator3/1
  findLeader/1(leader) -> Regular Vehicle Following/2(leader)
  Transfer Fcn/1 -> Gain/1
